simulink model "Cartesian_Regulation"  (R2022b)
settings: Solver=FixedStepAuto  StartTime=0.0  StopTime=50  MaxStep=0.1  RelTol=1e-3
undefined symbols (not defined in the file): unicycle, x_f, y_f
libraries: simulink_extras x1, dspsigops x1
settings Model: Creator=hp 2021  LastModifiedBy=Musta
settings OptimizationCC: EnhancedBackFolding=on  PassReuseOutputArgsAs=Individual arguments  ZeroExternalMemoryAtStartup=off  ZeroInternalMemoryAtStartup=off  MaxStackSize=64  OptimizeBlockOrder=speed  DifferentSizesBufferReuse=on  OptimizationCustomize=off  EfficientTunableParamExpr=on
settings DebuggingCC: ParameterTunabilityLossMsg=error
settings HardwareCC: ProdBitPerPointer=32  ProdBitPerSizeT=32  ProdBitPerPtrDiffT=32  ProdLargestAtomicFloat=None  ProdIntDivRoundTo=Undefined  ProdEndianess=Unspecified  ProdWordSize=32  ProdHWDeviceType=Generic->Unspecified (assume 32-bit Generic)
settings ModelReferenceCC: EnableRefExpFcnMdlSchedulingChecks=on
settings SFSimCC: MATLABDynamicMemAlloc=off
settings RTWCC: Description=Embedded Coder  SystemTargetFile=ert.tlc  HardwareBoard=Robot Operating System (ROS)  TLCOptions="-aInlineSetEventsForThisBaseRateFcn=TLC_FALSE -aSuppressMultiTaskScheduler=TLC_FALSE  -aRateBasedStepFcn=0"  TemplateMakefile=ert_default_tmf  Toolchain=Catkin  TargetLang=C++
settings CodeAppCC: ForceParamTrailComments=on  IgnoreCustomStorageClasses=off  OperatorAnnotations=on  SimulinkDataObjDesc=on  SFDataObjDesc=on  InsertBlockDesc=on

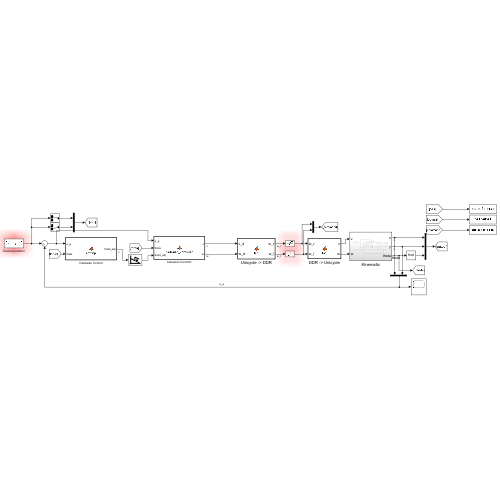
[thumbnail: Simulink's stored preview of the top-level diagram]
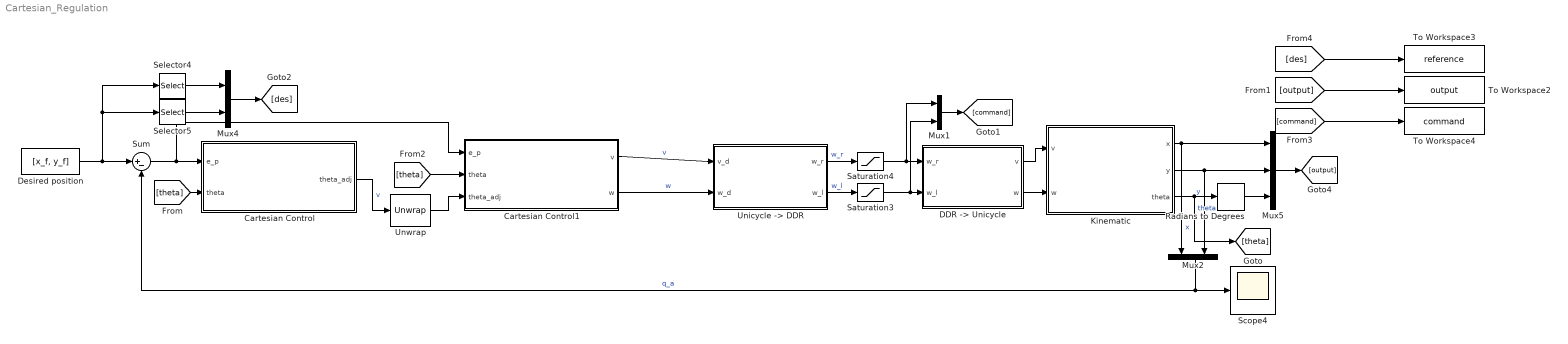
== system Cartesian_Regulation ==
  " DDR -> Unicycle " : MATLAB Function  TreatAsAtomicUnit=on
  Cartesian Control : MATLAB Function  TreatAsAtomicUnit=on
  Cartesian Control1 : MATLAB Function  TreatAsAtomicUnit=on
  Desired position : Constant  Value=[x_f, y_f]
  Kinematic : Subsystem
  Mux1 : Mux  Inputs=2
  Mux2 : Mux  Inputs=2
  Mux4 : Mux  Inputs=2
  Mux5 : Mux  Inputs=3
  Radians to Degrees : simulink_extras/Transformations/Radians to Degrees
  Saturation3 : Saturate  UpperLimit=unicycle.omegaWheelMax  LowerLimit=unicycle.omegaWheelMin
  Saturation4 : Saturate  UpperLimit=unicycle.omegaWheelMax  LowerLimit=unicycle.omegaWheelMin
  Scope4 : Scope
  Selector4 : Selector  InputPortWidth=2  IndexOptions=Index vector (dialog)  Indices=1  OutputSizes=1
  Selector5 : Selector  InputPortWidth=2  IndexOptions=Index vector (dialog)  Indices=2  OutputSizes=1
  Sum : Sum  Inputs=|+-
  To Workspace2 : ToWorkspace  VariableName=output  SaveFormat=Structure With Time  SampleTime=-1
  To Workspace3 : ToWorkspace  VariableName=reference  SaveFormat=Structure With Time  SampleTime=-1
  To Workspace4 : ToWorkspace  VariableName=command  SaveFormat=Structure With Time  SampleTime=-1
  "Unicycle -> DDR" : MATLAB Function  TreatAsAtomicUnit=on
  Unwrap : dspsigops/Unwrap  tol=0.99*pi  InputProcessing=Columns as channels (frame based)  running=off
  wires:
  Desired position/1 -> Selector4/1, Selector5/1, Sum/1
  Mux5/1 -> [output]
  Selector5/1 -> Mux4/2
  Selector4/1 -> Mux4/1
  [command] -> To Workspace4/1
  Radians to Degrees/1 -> Mux5/3
  Mux4/1 -> [des]
  [output] -> To Workspace2/1
  [des] -> To Workspace3/1
  Mux2/1 -> Sum/2, Scope4/1  "q_a"
  Sum/1 -> Cartesian Control1/1(e_p), Cartesian Control/1(e_p)
  " DDR -> Unicycle "/1(v) -> Kinematic/1(v)
  Kinematic/1(x) -> Mux5/1, Mux2/1  "x"
  "Unicycle -> DDR"/1(w_r) -> Saturation4/1  "w_r"
  Saturation4/1 -> Mux1/1, " DDR -> Unicycle "/1(w_r)
  Mux1/1 -> [command]
  "Unicycle -> DDR"/2(w_l) -> Saturation3/1  "w_l"
  Saturation3/1 -> Mux1/2, " DDR -> Unicycle "/2(w_l)
  Kinematic/3(theta) -> [theta], Radians to Degrees/1  "theta"
  " DDR -> Unicycle "/2(w) -> Kinematic/2(w)
  Kinematic/2(y) -> Mux5/2, Mux2/2  "y"
  [theta] -> Cartesian Control/2(theta)
  Cartesian Control1/1(v) -> "Unicycle -> DDR"/1(v_d)  "v"
  Cartesian Control1/2(w) -> "Unicycle -> DDR"/2(w_d)  "w"
  Cartesian Control/1(theta_adj) -> Unwrap/1  "v"
  Unwrap/1 -> Cartesian Control1/3(theta_adj)
  [theta] -> Cartesian Control1/2(theta)

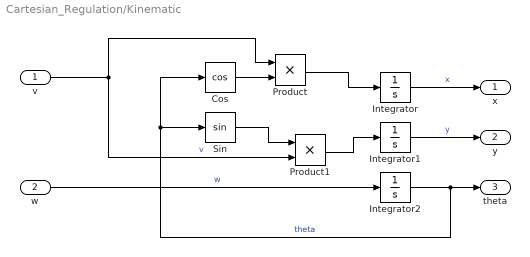
== system Cartesian_Regulation/Kinematic ==
  v : Inport
  w : Inport  Port=2
  Cos : Trigonometry  Operator=cos
  Integrator : Integrator  InitialCondition=unicycle.ic.x
  Integrator1 : Integrator  InitialCondition=unicycle.ic.y
  Integrator2 : Integrator  InitialCondition=unicycle.ic.theta
  Product : Product
  Product1 : Product
  Sin : Trigonometry
  x : Outport
  y : Outport  Port=2
  theta : Outport  Port=3
  wires:
  w/1 -> Integrator2/1  "w"
  Product/1 -> Integrator/1
  v/1 -> Product/1, Product1/2  "v"
  Cos/1 -> Product/2
  Integrator1/1 -> y/1  "y"
  Integrator/1 -> x/1  "x"
  Integrator2/1 -> Cos/1, Sin/1, theta/1  "theta"
  Product1/1 -> Integrator1/1
  Sin/1 -> Product1/1

== matlab function Cartesian_Regulation/Cartesian Control1 ==
  data: v output; w output; e_p input; theta input; theta_adj input
function [v,w] = cartesian_controller(e_p, theta, theta_adj)

    %#codegen
    coder.extrinsic('evalin')
    K_v = 0;                  % Needed in order to set variable class correctly
    K_w = 0;                  % Needed in order to set variable class correctly
    K_v = evalin('base','K_v'); % Read value from workspace
    K_w = evalin('base','K_w'); % Read value from workspace

    v = K_v * (e_p(1)*cos(theta) + e_p(2)*sin(theta));
%     p = atan2(e_p(2),e_p(1)) - theta;
%     % Count the number of turns around full circle
%     num_turns = floor(p/(2*pi));
%     % Adjust p to remove any full circle turns
%     theta_adj = p - num_turns*(2*pi);
    w = K_w * (theta_adj - theta);

end

== matlab function Cartesian_Regulation/Cartesian Control ==
  data: theta_adj output; e_p input; theta input
function theta_adj = unwrap(e_p, theta)

    theta_adj = mod(atan2(e_p(2),e_p(1)),2*pi);

end

== matlab function Cartesian_Regulation/ DDR -> Unicycle  ==
  data: w_r input; v output; w_l input; w output
function [v, w] = fcn(w_r, w_l)

    %#codegen
    coder.extrinsic('evalin')
    d = 0;                  % Needed in order to set variable class correctly
    r = 0;                  % Needed in order to set variable class correctly
    d = evalin('base','unicycle.d'); % Read value from workspace
    r = evalin('base','unicycle.r'); % Read value from workspace

    v = r*(w_r + w_l)/2; % rad/s
    w = r*(w_r - w_l)/d; % rad/s

end

== matlab function Cartesian_Regulation/Unicycle -> DDR ==
  data: v_d input; w_r output; w_d input; w_l output
function [w_r, w_l] = fcn(v_d, w_d)

    %#codegen
    coder.extrinsic('evalin')
    d = 0;                  % Needed in order to set variable class correctly
    r = 0;                  % Needed in order to set variable class correctly
    d = evalin('base','unicycle.d'); % Read value from workspace
    r = evalin('base','unicycle.r'); % Read value from workspace

    w_r = ((2 * v_d) + (w_d * d)) / (2 * r);
    w_l = ((2 * v_d) - (w_d * d)) / (2 * r);

end
